simulink model "Pacemaker_Group1"  (R2020a)
settings: Solver=FixedStepAuto  StartTime=0.0  StopTime=10.0  FixedStep=1e-3  RelTol=1e-3  EnableMultiTasking=on
undefined symbols (not defined in the file): D0, D1, D10, D11, D12, D13, D2, D3, D4, D5, D6, D7, D8, D9, PTA0, PTA1, PTA2, PTB23, PTB9, PTC16, PTC17, PTC2, PTC3, PTC4, PTD0, PTD1, PTD2, PTD3
libraries: frdmk64flib x17
settings Model: ExtModeTrigDuration=5  Creator=Luis  LastModifiedBy=Luis
settings OptimizationCC: EnhancedBackFolding=on  PassReuseOutputArgsAs=Individual arguments  ZeroExternalMemoryAtStartup=off  ZeroInternalMemoryAtStartup=off  MaxStackSize=64  OptimizeBlockOrder=speed  DifferentSizesBufferReuse=on  OptimizationCustomize=off  EfficientTunableParamExpr=on
settings DebuggingCC: ParameterTunabilityLossMsg=error
settings HardwareCC: ProdBitPerPointer=32  ProdBitPerSizeT=32  ProdBitPerPtrDiffT=32  ProdLargestAtomicInteger=Long  ProdLargestAtomicFloat=Double  ProdWordSize=32  ProdHWDeviceType=ARM Compatible->ARM Cortex
settings SFSimCC: MATLABDynamicMemAlloc=off
settings RTWCC: SystemTargetFile=ert.tlc  HardwareBoard=NXP FRDM-K64F  TemplateMakefile=ert_default_tmf  Toolchain=GNU Tools for ARM Embedded Processors
settings CodeAppCC: ForceParamTrailComments=on  IgnoreCustomStorageClasses=off  OperatorAnnotations=on  SimulinkDataObjDesc=on  SFDataObjDesc=on  InsertBlockDesc=on

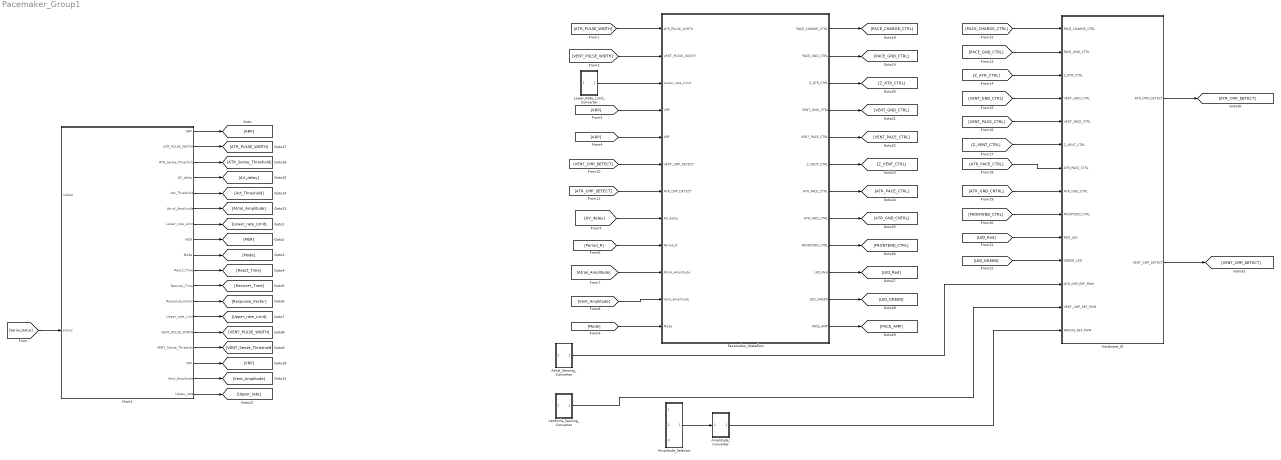
== system Pacemaker_Group1 ==
  Amplitude_Converter : Subsystem
  Amplitude_Selector : Subsystem
  Atrial_Sensing_Converter : Subsystem
  Chart1 : Stateflow chart  TreatAsAtomicUnit=on
  Hardware_IO : Subsystem
  Lower_Rate_Limit_Converter : Subsystem
  "Pacemaker_Stateflow " : Stateflow chart  TreatAsAtomicUnit=on
      settings: PortSchema="{\"entries\":[{\"content\":{\"sides\":[{\"content\":{\"connectorIds\":[\"In1\",\"In4\",\"In2\",\"In5\",\"In6\",\"In7\",\"In8\",\"In9\",\"In10\",\"In11\",\"In12\",\"In3\"]},\"type\":\"ConnectorPlacement.EquallySpacedRectSide\",\"uuid\":\"f97b12ff-cb00-4386-a373-7143c3a8b48d\"},{\"content\":{\"connectorIds\":[\"Out1\",\"Out2\",\"Out3\",\"Out4\",\"Out5\",\"Out6\",\"Out7\",\"Out8\",\"Out9\",\"Out10\",\"Out11\",\"Out12\"],\"side\":\"RIGHT\"},\"type\":\"ConnectorPlacement.EquallySpacedRectSide\",\"uuid\":\"90163773-f9d1-46de-bd72-9589b8539202\"},{\"content\":{\"connectorIds\":[],\"side\":\"TOP\"},\"type\":\"ConnectorPlacement.EquallySpacedRectSide\",\"uuid\":\"f8a54119-a7c4-4071-8260-df405210e670\"},{\"content\":{\"connectorIds\":[],\"side\":\"BOTTOM\"},\"type\":\"ConnectorPlacement.EquallySpacedRectSide\",\"uuid\":\"70f9d800-d0b8-46e1-812e-9f4712f7acbd\"}]},\"type\":\"ConnectorPlacement.EquallySpacedConnector\",\"uuid\":\"47f7c40c-c42b-42f7-beed-99d299c6cdee\"}],\"packageUris\":[\"http://schema.mathworks.com/mf0/Connector/19700101\"],\"version\":\"1.0\"}"
  Ventricle_Sensing_Converter : Subsystem
  wires:
  Lower_Rate_Limit_Converter/1(Out1) -> "Pacemaker_Stateflow "/2(Lower_rate_Limit)
  Amplitude_Selector/1(Out1) -> Amplitude_Converter/1(In1)
  Ventricle_Sensing_Converter/1(Out1) -> Hardware_IO/13(VENT_CMP_REF_PWM)
  Amplitude_Converter/1(Out1) -> Hardware_IO/14(PACING_REF_PWM)
  Atrial_Sensing_Converter/1(Out1) -> Hardware_IO/12(ATR_CMP_REF_PWM)
  Chart1/1(ARP) -> [ARP]
  Chart1/18(Upper_rate) -> [Upper_rate]
  Chart1/17(Vent_Amplitude) -> [Vent_Amplitude]
  Chart1/16(VRP) -> [VRP]
  Chart1/15(VENT_Sense_Threshold) -> [VENT_Sense_Threshold]
  Chart1/14(VENT_PULSE_WIDTH) -> [VENT_PULSE_WIDTH]
  Chart1/13(Upper_rate_Limit) -> [Upper_rate_Limit]
  Chart1/12(Response_Factor) -> [Response_Factor]
  Chart1/11(Recover_Time) -> [Recover_Time]
  Chart1/10(React_Time) -> [React_Time]
  Chart1/9(Mode) -> [Mode]
  Chart1/8(MSR) -> [MSR]
  Chart1/7(Lower_rate_Limit) -> [Lower_rate_Limit]
  Chart1/5(Act_Threshold) -> [Act_Threshold]
  Chart1/6(Atrial_Amplitude) -> [Atrial_Amplitude]
  Chart1/4(AV_delay) -> [AV_delay]
  Chart1/3(ATR_Sense_Threshold) -> [ATR_Sense_Threshold]
  Chart1/2(ATR_PULSE_WIDTH) -> [ATR_PULSE_WIDTH]
  [Serial_status] -> Chart1/2(status)
  [Mode] -> "Pacemaker_Stateflow "/3(Mode)
  [Vent_Amplitude] -> "Pacemaker_Stateflow "/12(Vent_Amplitude)
  [Atrial_Amplitude] -> "Pacemaker_Stateflow "/11(Atrial_Amplitude)
  [Period_R] -> "Pacemaker_Stateflow "/10(Period_R)
  [AV_delay] -> "Pacemaker_Stateflow "/9(AV_delay)
  [ARP] -> "Pacemaker_Stateflow "/6(ARP)
  [VRP] -> "Pacemaker_Stateflow "/5(VRP)
  [VENT_PULSE_WIDTH] -> "Pacemaker_Stateflow "/4(VENT_PULSE_WIDTH)
  [ATR_PULSE_WIDTH] -> "Pacemaker_Stateflow "/1(ATR_PULSE_WIDTH)
  [ATR_CMP_DETECT] -> "Pacemaker_Stateflow "/8(ATR_CMP_DETECT)
  [VENT_CMP_DETECT] -> "Pacemaker_Stateflow "/7(VENT_CMP_DETECT)
  "Pacemaker_Stateflow "/1(PACE_CHARGE_CTRL) -> [PACE_CHARGE_CTRL]
  "Pacemaker_Stateflow "/2(PACE_GND_CTRL) -> [PACE_GND_CTRL]
  "Pacemaker_Stateflow "/3(Z_ATR_CTRL) -> [Z_ATR_CTRL]
  "Pacemaker_Stateflow "/4(VENT_GND_CTRL) -> [VENT_GND_CTRL]
  "Pacemaker_Stateflow "/5(VENT_PACE_CTRL) -> [VENT_PACE_CTRL]
  "Pacemaker_Stateflow "/6(Z_VENT_CTRL) -> [Z_VENT_CTRL]
  "Pacemaker_Stateflow "/7(ATR_PACE_CTRL) -> [ATR_PACE_CTRL]
  "Pacemaker_Stateflow "/8(ATR_GND_CTRL) -> [ATR_GND_CNTRL]
  "Pacemaker_Stateflow "/9(FRONTEND_CTRL) -> [FRONTEND_CTRL]
  "Pacemaker_Stateflow "/10(LED_Red) -> [LED_Red]
  "Pacemaker_Stateflow "/11(LED_GREEN) -> [LED_GREEN]
  "Pacemaker_Stateflow "/12(PACE_AMP) -> [PACE_AMP]
  [PACE_CHARGE_CTRL] -> Hardware_IO/1(PACE_CHARGE_CTRL)
  [PACE_GND_CTRL] -> Hardware_IO/2(PACE_GND_CTRL)
  [Z_ATR_CTRL] -> Hardware_IO/3(Z_ATR_CTRL)
  [VENT_GND_CTRL] -> Hardware_IO/4(VENT_GND_CTRL)
  [VENT_PACE_CTRL] -> Hardware_IO/5(VENT_PACE_CTRL)
  [Z_VENT_CTRL] -> Hardware_IO/6(Z_VENT_CTRL)
  [ATR_PACE_CTRL] -> Hardware_IO/7(ATR_PACE_CTRL)
  [ATR_GND_CNTRL] -> Hardware_IO/8(ATR_GND_CTRL)
  [FRONTEND_CTRL] -> Hardware_IO/9(FRONTEND_CTRL)
  [LED_Red] -> Hardware_IO/10(RED_LED)
  [LED_GREEN] -> Hardware_IO/11(GREEN_LED)
  Hardware_IO/1(ATR_CMP_DETECT) -> [ATR_CMP_DETECT]
  Hardware_IO/2(VENT_CMP_DETECT) -> [VENT_CMP_DETECT]

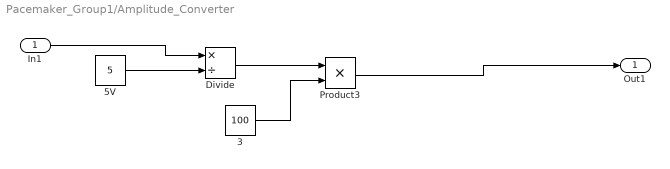
== system Pacemaker_Group1/Amplitude_Converter ==
  In1 : Inport
  3 : Constant  Value=100  OutDataTypeStr=double
  5V : Constant  Value=5  OutDataTypeStr=double
  Divide : Product  Inputs=*/  OutDataTypeStr=double  RndMeth=Nearest
  Product3 : Product  OutDataTypeStr=double
  Out1 : Outport
  wires:
  Product3/1 -> Out1/1
  3/1 -> Product3/2
  In1/1 -> Divide/1
  Divide/1 -> Product3/1
  5V/1 -> Divide/2

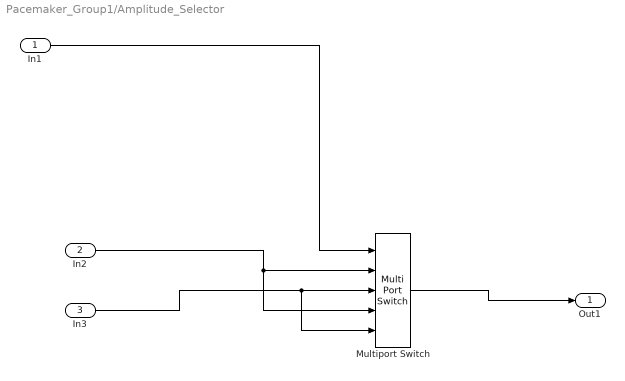
== system Pacemaker_Group1/Amplitude_Selector ==
  In1 : Inport
  In2 : Inport  Port=2
  In3 : Inport  Port=3
  Multiport Switch : MultiPortSwitch  DataPortOrder=Zero-based contiguous  Inputs=4  zeroidx=on  OutDataTypeStr=double
  Out1 : Outport
  wires:
  Multiport Switch/1 -> Out1/1
  In3/1 -> Multiport Switch/5, Multiport Switch/3
  In1/1 -> Multiport Switch/1
  In2/1 -> Multiport Switch/4, Multiport Switch/2

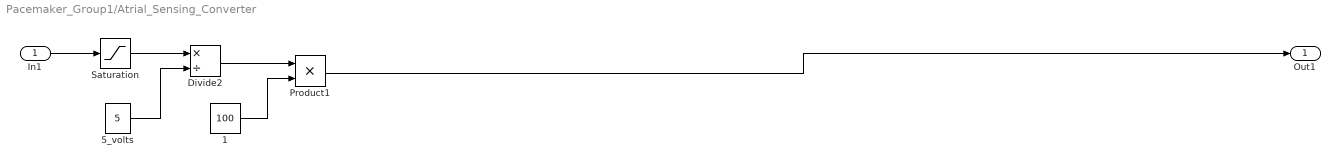
== system Pacemaker_Group1/Atrial_Sensing_Converter ==
  In1 : Inport
  1 : Constant  Value=100  OutDataTypeStr=uint16
  5_volts : Constant  Value=5  OutDataTypeStr=double
  Divide2 : Product  Inputs=*/
  Product1 : Product  OutDataTypeStr=uint16
  Saturation : Saturate  UpperLimit=4  LowerLimit=0.65  LinearizeAsGain=off  OutDataTypeStr=double
  Out1 : Outport
  wires:
  Product1/1 -> Out1/1
  1/1 -> Product1/2
  Divide2/1 -> Product1/1
  5_volts/1 -> Divide2/2
  In1/1 -> Saturation/1
  Saturation/1 -> Divide2/1

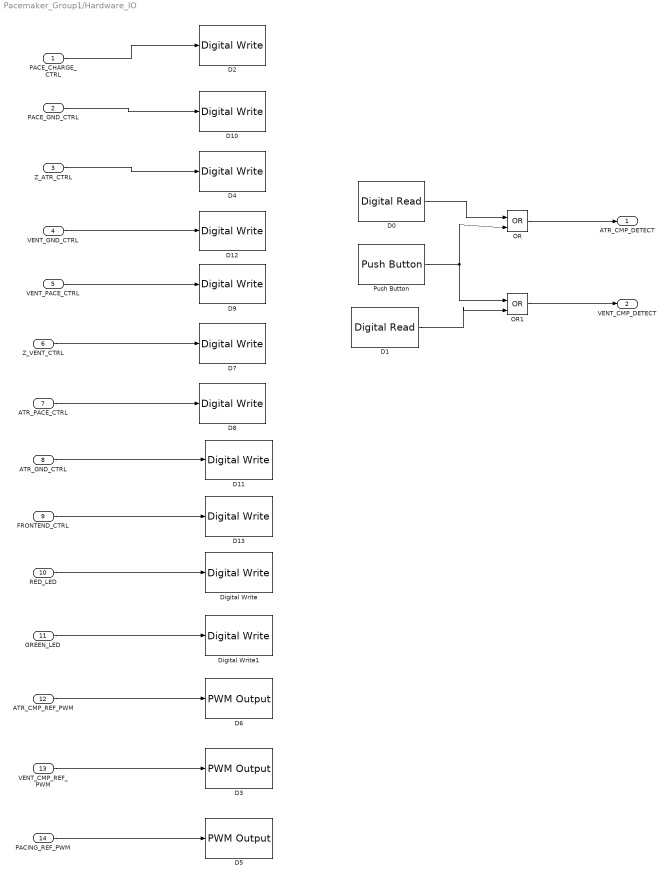
== system Pacemaker_Group1/Hardware_IO ==
  PACE_CHARGE_CTRL : Inport
  PACE_GND_CTRL : Inport  Port=2
  Z_ATR_CTRL : Inport  Port=3
  VENT_GND_CTRL : Inport  Port=4
  VENT_PACE_CTRL : Inport  Port=5
  Z_VENT_CTRL : Inport  Port=6
  ATR_PACE_CTRL : Inport  Port=7
  ATR_GND_CTRL : Inport  Port=8
  FRONTEND_CTRL : Inport  Port=9
  RED_LED : Inport  Port=10
  GREEN_LED : Inport  Port=11
  ATR_CMP_REF_PWM : Inport  Port=12
  VENT_CMP_REF_PWM : Inport  Port=13
  PACING_REF_PWM : Inport  Port=14
  D0 : frdmk64flib/Digital Read  Whichpin=PTC16 (D0)  SampleTime=-1
  D1 : frdmk64flib/Digital Read  Whichpin=PTC17 (D1)  SampleTime=-1
  D10 : frdmk64flib/Digital Write  Whichpin=PTD0 (D10)
  D11 : frdmk64flib/Digital Write  Whichpin=PTD2 (D11)
  D12 : frdmk64flib/Digital Write  Whichpin=PTD3 (D12)
  D13 : frdmk64flib/Digital Write  Whichpin=PTD1 (D13)
  D2 : frdmk64flib/Digital Write  Whichpin=PTB9 (D2)
  D3 : frdmk64flib/PWM Output  Whichpin=PTA1 (D3)  InitialFrequency=2000  InitialDutyCycle=0
  D4 : frdmk64flib/Digital Write  Whichpin=PTB23 (D4)
  D5 : frdmk64flib/PWM Output  Whichpin=PTA2 (D5)  InitialFrequency=2000  InitialDutyCycle=0
  D6 : frdmk64flib/PWM Output  Whichpin=PTC2 (D6)  InitialFrequency=2000  InitialDutyCycle=0
  D7 : frdmk64flib/Digital Write  Whichpin=PTC3 (D7)
  D8 : frdmk64flib/Digital Write  Whichpin=PTA0 (D8)
  D9 : frdmk64flib/Digital Write  Whichpin=PTC4 (D9)
  Digital Write : frdmk64flib/Digital Write  Whichpin=RED_LED
  Digital Write1 : frdmk64flib/Digital Write  Whichpin=GREEN_LED
  OR : Logic  Operator=OR  IconShape=distinctive  AllPortsSameDT=off  OutDataTypeStr=boolean
  OR1 : Logic  Operator=OR  IconShape=distinctive  AllPortsSameDT=off  OutDataTypeStr=boolean
  Push Button : frdmk64flib/Push Button  Whichswitch=SW2  SampleTime1=-1
  ATR_CMP_DETECT : Outport
  VENT_CMP_DETECT : Outport  Port=2
  wires:
  PACING_REF_PWM/1 -> D5/1
  RED_LED/1 -> Digital Write/1
  Z_ATR_CTRL/1 -> D4/1
  PACE_CHARGE_CTRL/1 -> D2/1
  VENT_GND_CTRL/1 -> D12/1
  D1/1 -> OR1/2
  ATR_PACE_CTRL/1 -> D8/1
  OR1/1 -> VENT_CMP_DETECT/1
  PACE_GND_CTRL/1 -> D10/1
  ATR_GND_CTRL/1 -> D11/1
  OR/1 -> ATR_CMP_DETECT/1
  D0/1 -> OR/1
  ATR_CMP_REF_PWM/1 -> D6/1
  Push Button/1 -> OR1/1, OR/2
  GREEN_LED/1 -> Digital Write1/1
  FRONTEND_CTRL/1 -> D13/1
  VENT_CMP_REF_PWM/1 -> D3/1
  Z_VENT_CTRL/1 -> D7/1
  VENT_PACE_CTRL/1 -> D9/1

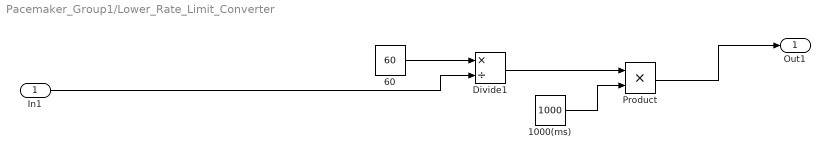
== system Pacemaker_Group1/Lower_Rate_Limit_Converter ==
  In1 : Inport
  1000(ms) : Constant  Value=1000  OutDataTypeStr=uint16
  60 : Constant  Value=60  OutDataTypeStr=uint16
  Divide1 : Product  Inputs=*/
  Product : Product  OutDataTypeStr=uint16
  Out1 : Outport
  wires:
  60/1 -> Divide1/1
  In1/1 -> Divide1/2
  Product/1 -> Out1/1
  Divide1/1 -> Product/1
  1000(ms)/1 -> Product/2

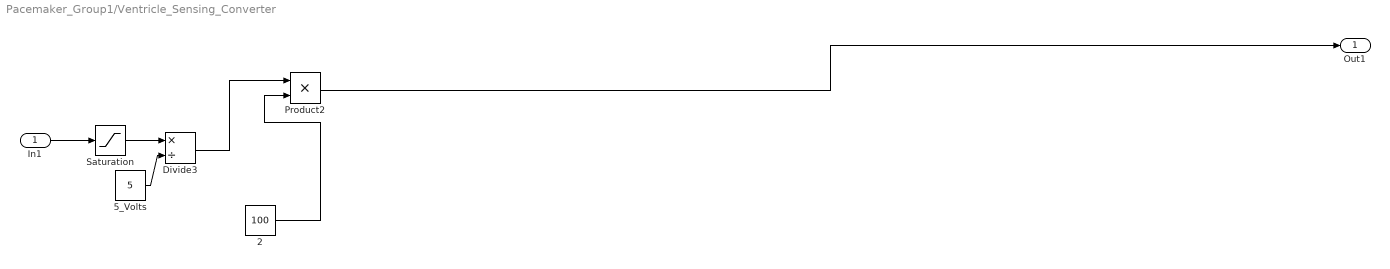
== system Pacemaker_Group1/Ventricle_Sensing_Converter ==
  In1 : Inport
  2 : Constant  Value=100  OutDataTypeStr=uint16
  5_Volts : Constant  Value=5  OutDataTypeStr=double
  Divide3 : Product  Inputs=*/
  Product2 : Product  OutDataTypeStr=uint16
  Saturation : Saturate  UpperLimit=4  LowerLimit=0.65  OutDataTypeStr=double
  Out1 : Outport
  wires:
  Product2/1 -> Out1/1
  5_Volts/1 -> Divide3/2
  Divide3/1 -> Product2/1
  In1/1 -> Saturation/1
  2/1 -> Product2/2
  Saturation/1 -> Divide3/1

== stateflow chart Pacemaker_Group1/Chart1 ==
  state PARAMETER_CHECK
    entry:
    if Lower_rate_Limit < 50 || Lower_rate_Limit > 175||Upper_rate_Limit < 75 || Upper_rate >175 ...
    || Atrial_Amplitude < 0.5 || Atrial_Amplitude > 5 || Vent_Amplitude < 0.5 || Vent_Amplitude > 5 ...
    || ATR_PULSE_WIDTH < 1 || ATR_PULSE_WIDTH > 10 || VENT_PULSE_WIDTH < 1 || VENT_PULSE_WIDTH > 10 ...
    || ATR_Sense_Threshold < 0.5 || ATR_Sense_Threshold > 3.3 || VENT_Sense_Threshold < 0.5 || VENT_Sense_Threshold > 3.3 ...
    || ARP < 150 || ARP > 500 || VRP < 150 || VRP > 500 ...
    || AV_delay < 70 || AV_delay > 300 || React_Time < 1 || React_Time > 30 ...
    || Recover_Time < 5 ||  Recover_Time > 30 || Response_Factor < 1 || Response_Factor > 16 ...
    || Act_Threshold < 1 || Act_Threshold > 4 || MSR < 50 || MSR > 175 ...
    end
  state SET_PARAMS
    entry:
    Mode = rxdata(2);
    Lower_rate_Limit=typecast(rxdata(3:4), 'unit16');
    Upper_rate_Limit=typecast(rxdata(5:6), 'unit16');
    Atrial_Amplitude=typecast(rxdata(7:14), 'double');
    Vent_Amplitude=typecast(rxdata(15:22), 'double');
    ATR_PULSE_WIDTH=typecast(rxdata(22:23), 'unit16');
    VENT_PULSE_WIDTH=typecast(rxdata(24:25), 'unit16');
    ATR_Sense_Threshold=typecast(rxdata(26:33), 'double');
    VENT_Sense_Threshold=typecast(rxdata(34:41), 'double');
    ARP=typecast(rxdata(42:43), 'unit16');
    VRP=typecast(rxdata(44:45), 'unit16');
    AV_delay=typecast(rxdata(46:47), 'unit16');
    React_Time=typecast(rxdata(48:49), 'unit16');
    Recover_Time=typecast(rxdata(50:51), 'unit16');
    Response_Factor=8;
    Act_Threshold=1;
    MSR=120;
    send_params();
  state INTIAL
    entry:
    Mode = 0;
    Lower_rate_Limit=60;
    Atrial_Amplitude=3.3;
    Vent_Amplitude=3.3;
    ATR_PULSE_WIDTH=10;
    VENT_PULSE_WIDTH=10;
    ATR_Sense_Threshold=2.75;
    VENT_Sense_Threshold=2.75;
    ARP=300;
    VRP=300;
    AV_delay=100;
    React_Time=30;
    Recover_Time=5;
    Response_Factor=8;
    Act_Threshold=1;
    MSR=120;
  state STANBY
    %Waiting for COM
  state EGRAM
    entry:
    send_params();
  SET_PARAMS -> PARAMETER_CHECK
  PARAMETER_CHECK -> STANBY
  (junction 11) -> SET_PARAMS [order 1] : [rxdata(1) == hex2dec(55)]
  (default) -> INTIAL
  STANBY -> (junction 11) : [status ==0 ]
  (junction 11) -> STANBY [order 3]
  (junction 11) -> EGRAM [order 2] : [rxdata(1) == hex2dec(22)]
  INTIAL -> STANBY
  data: rxdata input uint8; ARP output uint16; ATR_PULSE_WIDTH output single; ATR_Sense_Threshold output uint16; status input uint8; AV_delay output uint16; Act_Threshold output uint8; Atrial_Amplitude output uint16; Lower_rate_Limit output uint16; MSR output uint16; Mode output uint8; React_Time output uint16; Recover_Time output uint16; Response_Factor output uint8; Upper_rate_Limit output uint16; VENT_PULSE_WIDTH output single; VENT_Sense_Threshold output uint16; VRP output uint16; Vent_Amplitude output uint16; Upper_rate output

== stateflow chart Pacemaker_Group1/Pacemaker_Stateflow  ==
  state AOO
    state AOO_CHARGING
      entry:
      %Charge C22
      ATR_PACE_CTRL=false;
      VENT_PACE_CTRL=false;
      PACE_CHARGE_CTRL=true;
      %Discharge C21
      PACE_GND_CTRL=true;
      Z_VENT_CTRL=false;
      Z_ATR_CTRL=false;
      ATR_GND_CTRL=true;
      VENT_GND_CTRL=false;
      LED_Red = false;
    state AOO_DISCHARGING
      entry:
      %Discharge C22 into ATR
      %Charge C21
      PACE_CHARGE_CTRL=false;
      PACE_GND_CTRL=true;
      ATR_PACE_CTRL=true;
      ATR_GND_CTRL=false;
      Z_VENT_CTRL=false;
      Z_ATR_CTRL=false;
      VENT_GND_CTRL=false;
      VENT_PACE_CTRL=false;
      LED_Red = true;
    AOO_DISCHARGING -> AOO_CHARGING : after(ATR_PULSE_WIDTH,msec)
    AOO_CHARGING -> AOO_DISCHARGING [order 1] : after(Lower_rate_Limit - ATR_PULSE_WIDTH,msec)
  state DOOR [group]
    state DOOR_CHARGING_V
      entry:
      %Charge C22
      VENT_PACE_CTRL=false;
      ATR_PACE_CTRL=false;
      PACE_CHARGE_CTRL=true;
      %Discharge C21 to V
      PACE_GND_CTRL=true;
      Z_VENT_CTRL=false;
      Z_ATR_CTRL=false;
      ATR_PACE_CTRL=false;
      ATR_GND_CTRL=false;
      VENT_GND_CTRL=true;
      LED_GREEN = false;
      %Set PACING_REF_PWM
      PACE_AMP=Atrial_Amplitude;
    state DOOR_PACE_A
      entry:
      %Discharge C22 into ATR
      %Charge C21
      PACE_CHARGE_CTRL=false;
      PACE_GND_CTRL=true;
      ATR_PACE_CTRL=true;
      ATR_GND_CTRL=false;
      Z_VENT_CTRL=false;
      Z_ATR_CTRL=false;
      VENT_GND_CTRL=false;
      VENT_PACE_CTRL=false;
      LED_Red = true;
    state DOOR_CHARGING_A
      entry:
      %Charge C22
      ATR_PACE_CTRL=false;
      VENT_PACE_CTRL=false;
      PACE_CHARGE_CTRL=true;
      %Discharge C21
      PACE_GND_CTRL=true;
      Z_VENT_CTRL=false;
      Z_ATR_CTRL=false;
      ATR_GND_CTRL=true;
      VENT_GND_CTRL=false;
      LED_Red = false;
      %Set PACING_REF_PWM
      PACE_AMP=Vent_Amplitude
    state DOOR_PACE_V
      entry:
      %Discharge C22 into VENT
      %Charge C21
      PACE_CHARGE_CTRL=false;
      PACE_GND_CTRL=true;
      ATR_PACE_CTRL=false;
      ATR_GND_CTRL=false;
      Z_ATR_CTRL=false
      Z_VENT_CTRL=false;
      VENT_GND_CTRL=false;
      VENT_PACE_CTRL=true;
      LED_GREEN = true;
    DOOR_CHARGING_V -> DOOR_PACE_A [order 1] : after(Period_R - (AV_delay+VENT_PULSE_WIDTH),msec)
    DOOR_PACE_A -> DOOR_CHARGING_A : after(ATR_PULSE_WIDTH,msec)
    DOOR_PACE_V -> DOOR_CHARGING_V : after(VENT_PULSE_WIDTH, msec)
    DOOR_CHARGING_A -> DOOR_PACE_V : after(AV_delay - ATR_PULSE_WIDTH,msec)
  state VOO [group]
    state VOO_DISCHARGE
      entry:
      %Discharge C22 into VENT
      %Charge C21
      PACE_CHARGE_CTRL=false;
      PACE_GND_CTRL=true;
      ATR_PACE_CTRL=false;
      ATR_GND_CTRL=false;
      Z_ATR_CTRL=false
      Z_VENT_CTRL=false;
      VENT_GND_CTRL=false;
      VENT_PACE_CTRL=true;
      LED_GREEN = true;
    state VOO_CHARGING
      entry:
      %Charge C22
      VENT_PACE_CTRL=false;
      ATR_PACE_CTRL=false;
      PACE_CHARGE_CTRL=true;
      %Discharge C21
      PACE_GND_CTRL=true;
      Z_VENT_CTRL=false;
      Z_ATR_CTRL=false;
      ATR_PACE_CTRL=false;
      ATR_GND_CTRL=false;
      VENT_GND_CTRL=true;
      LED_GREEN = false;
    VOO_DISCHARGE -> VOO_CHARGING : after(VENT_PULSE_WIDTH, msec)
    VOO_CHARGING -> VOO_DISCHARGE [order 1] : after(Lower_rate_Limit - VENT_PULSE_WIDTH, msec)
  state VVIR [group]
    state CHARGING_C22
      entry:
      FRONTEND_CTRL = true;
      PACE_GND_CTRL = true;
      VENT_PACE_CTRL=false;
      ATR_PACE_CTRL=false;
      PACE_CHARGE_CTRL=true;
      Z_VENT_CTRL=false;
      Z_ATR_CTRL=false;
      ATR_GND_CTRL=false;
      VENT_GND_CTRL=true;
      LED_GREEN = false;
    state VENTRICAL_PACE
      entry:
      FRONTEND_CTRL = false;
      PACE_GND_CTRL = true;
      VENT_PACE_CTRL=true;
      ATR_PACE_CTRL=false;
      PACE_CHARGE_CTRL=false;
      Z_VENT_CTRL=false;
      Z_ATR_CTRL=false;
      ATR_GND_CTRL=false;
      VENT_GND_CTRL=false;
      LED_GREEN = true;
    state VRP_State
      entry:
      PACE_GND_CTRL = true;
      VENT_PACE_CTRL=false;
      ATR_PACE_CTRL=false;
      PACE_CHARGE_CTRL=true;
      Z_VENT_CTRL=false;
      Z_ATR_CTRL=false;
      ATR_GND_CTRL=false;
      VENT_GND_CTRL=true;
      LED_GREEN = false;
    VVIR.CHARGING_C22 -> VVIR.VENTRICAL_PACE [order 2] : after(Period_R - (VENT_PULSE_WIDTH + VRP), msec)
    VVIR.CHARGING_C22 -> VVIR.VRP_State [order 1] : [VENT_CMP_DETECT == true]
    VVIR.VRP_State -> VVIR.CHARGING_C22 : after(VRP, msec)
    VVIR.VENTRICAL_PACE -> VVIR.VRP_State : after(VENT_PULSE_WIDTH, msec)
  state VVI [group]
    state CHARGING_C22
      entry:
      FRONTEND_CTRL = true;
      PACE_GND_CTRL = true;
      VENT_PACE_CTRL=false;
      ATR_PACE_CTRL=false;
      PACE_CHARGE_CTRL=true;
      Z_VENT_CTRL=false;
      Z_ATR_CTRL=false;
      ATR_GND_CTRL=false;
      VENT_GND_CTRL=true;
      LED_GREEN = false;
    state VENTRICAL_PACE
      entry:
      FRONTEND_CTRL = false;
      PACE_GND_CTRL = true;
      VENT_PACE_CTRL=true;
      ATR_PACE_CTRL=false;
      PACE_CHARGE_CTRL=false;
      Z_VENT_CTRL=false;
      Z_ATR_CTRL=false;
      ATR_GND_CTRL=false;
      VENT_GND_CTRL=false;
      LED_GREEN = true;
    state VRP_State
      entry:
      PACE_GND_CTRL = true;
      VENT_PACE_CTRL=false;
      ATR_PACE_CTRL=false;
      PACE_CHARGE_CTRL=true;
      Z_VENT_CTRL=false;
      Z_ATR_CTRL=false;
      ATR_GND_CTRL=false;
      VENT_GND_CTRL=true;
      LED_GREEN = false;
    VVI.CHARGING_C22 -> VVI.VENTRICAL_PACE [order 2] : after((Lower_rate_Limit) - (VENT_PULSE_WIDTH + VRP), msec)
    VVI.CHARGING_C22 -> VVI.VRP_State [order 1] : [VENT_CMP_DETECT == true]
    VVI.VRP_State -> VVI.CHARGING_C22 : after(VRP, msec)
    VVI.VENTRICAL_PACE -> VVI.VRP_State : after(VENT_PULSE_WIDTH, msec)
  state Default
    entry:
    %Charge C22
    ATR_PACE_CTRL=false;
    VENT_PACE_CTRL=false;
    PACE_CHARGE_CTRL=false;
    %Discharge C21
    PACE_GND_CTRL=false;
    Z_VENT_CTRL=false;
    Z_ATR_CTRL=false;
    ATR_GND_CTRL=false;
    VENT_GND_CTRL=false;
    FRONTEND_CTRL=true;
    LED_Red=true;
    LED_GREEN=false;
  state AAIR [group]
    state CHARGING_C22
      entry:
      FRONTEND_CTRL = true;
      PACE_GND_CTRL = true;
      VENT_PACE_CTRL=false;
      ATR_PACE_CTRL=false;
      PACE_CHARGE_CTRL=true;
      Z_VENT_CTRL=false;
      Z_ATR_CTRL=false;
      ATR_GND_CTRL=true;
      VENT_GND_CTRL=false;
      LED_Red = false;
    state ATRIAL_PACE
      entry:
      FRONTEND_CTRL = false;
      PACE_GND_CTRL = true;
      VENT_PACE_CTRL=false;
      ATR_PACE_CTRL=true;
      PACE_CHARGE_CTRL=false;
      Z_VENT_CTRL=false;
      Z_ATR_CTRL=false;
      ATR_GND_CTRL=false;
      VENT_GND_CTRL=false;
      LED_Red = true;
    state ARP_State
      entry:
      PACE_GND_CTRL = true;
      VENT_PACE_CTRL=false;
      ATR_PACE_CTRL=false;
      PACE_CHARGE_CTRL=true;
      Z_VENT_CTRL=false;
      Z_ATR_CTRL=false;
      ATR_GND_CTRL=true;
      VENT_GND_CTRL=false;
      LED_Red = false;
    AAIR.CHARGING_C22 -> AAIR.ATRIAL_PACE [order 2] : after((Period_R) - (ATR_PULSE_WIDTH + ARP), msec)
    AAIR.CHARGING_C22 -> AAIR.ARP_State [order 1] : [ATR_CMP_DETECT == true]
    AAIR.ARP_State -> AAIR.CHARGING_C22 : after(ARP, msec)
    AAIR.ATRIAL_PACE -> AAIR.ARP_State : after(ATR_PULSE_WIDTH, msec)
  state AAI [group]
    state CHARGING_C22
      entry:
      FRONTEND_CTRL = true;
      PACE_GND_CTRL = true;
      VENT_PACE_CTRL=false;
      ATR_PACE_CTRL=false;
      PACE_CHARGE_CTRL=true;
      Z_VENT_CTRL=false;
      Z_ATR_CTRL=false;
      ATR_GND_CTRL=true;
      VENT_GND_CTRL=false;
      LED_Red = false;
    state ATRIAL_PACE
      entry:
      FRONTEND_CTRL = false;
      PACE_GND_CTRL = true;
      VENT_PACE_CTRL=false;
      ATR_PACE_CTRL=true;
      PACE_CHARGE_CTRL=false;
      Z_VENT_CTRL=false;
      Z_ATR_CTRL=false;
      ATR_GND_CTRL=false;
      VENT_GND_CTRL=false;
      LED_Red = true;
    state ARP_State
      entry:
      PACE_GND_CTRL = true;
      VENT_PACE_CTRL=false;
      ATR_PACE_CTRL=false;
      PACE_CHARGE_CTRL=true;
      Z_VENT_CTRL=false;
      Z_ATR_CTRL=false;
      ATR_GND_CTRL=true;
      VENT_GND_CTRL=false;
      LED_Red = false;
    AAI.CHARGING_C22 -> AAI.ATRIAL_PACE [order 2] : after((Lower_rate_Limit) - (ATR_PULSE_WIDTH + ARP), msec)
    AAI.CHARGING_C22 -> AAI.ARP_State [order 1] : [ATR_CMP_DETECT == true]
    AAI.ARP_State -> AAI.CHARGING_C22 : after(ARP, msec)
    AAI.ATRIAL_PACE -> AAI.ARP_State : after(ATR_PULSE_WIDTH, msec)
  state VOOR [group]
    state VOOR_DISCHARGE
      entry:
      %Discharge C22 into VENT
      %Charge C21
      PACE_CHARGE_CTRL=false;
      PACE_GND_CTRL=true;
      ATR_PACE_CTRL=false;
      ATR_GND_CTRL=false;
      Z_ATR_CTRL=false
      Z_VENT_CTRL=false;
      VENT_GND_CTRL=false;
      VENT_PACE_CTRL=true;
      LED_GREEN = true;
    state VOOR_CHARGING
      entry:
      %Charge C22
      VENT_PACE_CTRL=false;
      ATR_PACE_CTRL=false;
      PACE_CHARGE_CTRL=true;
      %Discharge C21
      PACE_GND_CTRL=true;
      Z_VENT_CTRL=false;
      Z_ATR_CTRL=false;
      ATR_PACE_CTRL=false;
      ATR_GND_CTRL=false;
      VENT_GND_CTRL=true;
      LED_GREEN = false;
    VOOR_DISCHARGE -> VOOR_CHARGING : after(VENT_PULSE_WIDTH, msec)
    VOOR_CHARGING -> VOOR_DISCHARGE [order 1] : after(Period_R - VENT_PULSE_WIDTH, msec)
  state DOO [group]
    state DOO_CHARGING_V
      entry:
      %Charge C22
      VENT_PACE_CTRL=false;
      ATR_PACE_CTRL=false;
      PACE_CHARGE_CTRL=true;
      %Discharge C21 to V
      PACE_GND_CTRL=true;
      Z_VENT_CTRL=false;
      Z_ATR_CTRL=false;
      ATR_PACE_CTRL=false;
      ATR_GND_CTRL=false;
      VENT_GND_CTRL=true;
      LED_GREEN = false;
      %Set PACING_REF_PWM
      PACE_AMP=Atrial_Amplitude;
    state DOO_PACE_A
      entry:
      %Discharge C22 into ATR
      %Charge C21
      PACE_CHARGE_CTRL=false;
      PACE_GND_CTRL=true;
      ATR_PACE_CTRL=true;
      ATR_GND_CTRL=false;
      Z_VENT_CTRL=false;
      Z_ATR_CTRL=false;
      VENT_GND_CTRL=false;
      VENT_PACE_CTRL=false;
      LED_Red = true;
    state DOO_CHARGING_A
      entry:
      %Charge C22
      ATR_PACE_CTRL=false;
      VENT_PACE_CTRL=false;
      PACE_CHARGE_CTRL=true;
      %Discharge C21
      PACE_GND_CTRL=true;
      Z_VENT_CTRL=false;
      Z_ATR_CTRL=false;
      ATR_GND_CTRL=true;
      VENT_GND_CTRL=false;
      LED_Red = false;
      %Set PACING_REF_PWM
      PACE_AMP=Vent_Amplitude
    state DOO_PACE_V
      entry:
      %Discharge C22 into VENT
      %Charge C21
      PACE_CHARGE_CTRL=false;
      PACE_GND_CTRL=true;
      ATR_PACE_CTRL=false;
      ATR_GND_CTRL=false;
      Z_ATR_CTRL=false
      Z_VENT_CTRL=false;
      VENT_GND_CTRL=false;
      VENT_PACE_CTRL=true;
      LED_GREEN = true;
    DOO_CHARGING_V -> DOO_PACE_A [order 1] : after(Lower_rate_Limit-(AV_delay+VENT_PULSE_WIDTH),msec)
    DOO_PACE_A -> DOO_CHARGING_A : after(ATR_PULSE_WIDTH,msec)
    DOO_PACE_V -> DOO_CHARGING_V : after(VENT_PULSE_WIDTH, msec)
    DOO_CHARGING_A -> DOO_PACE_V : after(AV_delay - ATR_PULSE_WIDTH,msec)
  state AOOR
    state AOOR_DISCHARGING
      entry:
      %Discharge C22 into ATR
      %Charge C21
      PACE_CHARGE_CTRL=false;
      PACE_GND_CTRL=true;
      ATR_PACE_CTRL=true;
      ATR_GND_CTRL=false;
      Z_VENT_CTRL=false;
      Z_ATR_CTRL=false;
      VENT_GND_CTRL=false;
      VENT_PACE_CTRL=false;
      LED_Red = true;
    state AOOR_CHARGING
      entry:
      %Charge C22
      ATR_PACE_CTRL=false;
      VENT_PACE_CTRL=false;
      PACE_CHARGE_CTRL=true;
      %Discharge C21
      PACE_GND_CTRL=true;
      Z_VENT_CTRL=false;
      Z_ATR_CTRL=false;
      ATR_GND_CTRL=true;
      VENT_GND_CTRL=false;
      LED_Red = false;
    (default) -> AOOR_CHARGING
    AOOR_CHARGING -> AOOR_DISCHARGING [order 1] : after(Period_R - ATR_PULSE_WIDTH,msec)
    AOOR_DISCHARGING -> AOOR_CHARGING : after(ATR_PULSE_WIDTH,msec)
  Default -> DOOR_CHARGING_V [order 8] : [Mode == 10]
  DOOR_CHARGING_V -> Default [order 2] : [Mode~=10]
  Default -> AOO_CHARGING [order 1] : [Mode == 1]
  AOO_CHARGING -> Default [order 2] : [Mode~=1]
  Default -> VOO_CHARGING [order 2] : [Mode == 2]
  VOO_CHARGING -> Default [order 2] : [Mode~=2]
  Default -> VVIR.CHARGING_C22 [order 9] : [Mode ==9]
  VVIR.CHARGING_C22 -> Default [order 3] : [Mode ~= 9]
  Default -> VVI.CHARGING_C22 [order 3] : [Mode == 3]
  VVI.CHARGING_C22 -> Default [order 3] : [Mode ~= 3]
  (default) -> Default
  Default -> AAIR.CHARGING_C22 [order 10] : [Mode == 8]
  AAIR.CHARGING_C22 -> Default [order 3] : [Mode ~= 8]
  Default -> AAI.CHARGING_C22 [order 4] : [Mode == 4]
  AAI.CHARGING_C22 -> Default [order 3] : [Mode ~= 4]
  Default -> VOOR_CHARGING [order 7] : [Mode == 7]
  VOOR_CHARGING -> Default [order 2] : [Mode ~= 7]
  Default -> AOOR_CHARGING [order 6] : [Mode == 6]
  AOOR_CHARGING -> Default [order 2] : [Mode ~=6]
  DOO_CHARGING_V -> Default [order 2] : [Mode ~= 5]
  Default -> DOO_CHARGING_V [order 5] : [Mode == 5]
  data: PACE_CHARGE_CTRL output boolean; PACE_GND_CTRL output boolean; Z_ATR_CTRL output boolean; VENT_GND_CTRL output boolean; VENT_PACE_CTRL output boolean; Z_VENT_CTRL output boolean; ATR_PULSE_WIDTH input uint16; Lower_rate_Limit input uint16; Mode input uint8; ATR_PACE_CTRL output boolean; ATR_GND_CTRL output boolean; VENT_PULSE_WIDTH input uint16; VRP input uint16; ARP input uint16; FRONTEND_CTRL output boolean; VENT_CMP_DETECT input boolean; ATR_CMP_DETECT input boolean; LED_Red output boolean; LED_GREEN output boolean; AV_delay input uint16; Period_R input uint16; Atrial_Amplitude input double; Vent_Amplitude input double; PACE_AMP output double
